simulink model "Test_OmniTorque_Lib"  (Simulink 7.6)
settings: Solver=ode3  StartTime=0.0  StopTime=inf  RelTol=1e-3
libraries: PhanTorque_3Dof_Library_32Bits x6
settings Model: Creator=carlos.aldana  LastModifiedBy=carlos.aldana
settings DebuggingCC: CheckSSInitialOutputMsg=off

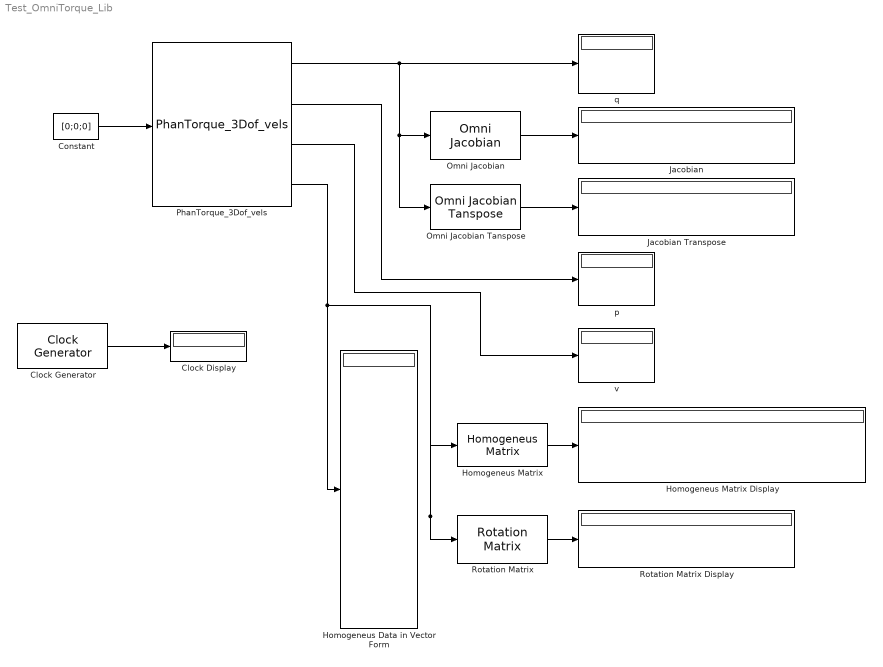
== system Test_OmniTorque_Lib ==
  Clock Display : Display
  Clock Generator : PhanTorque_3Dof_Library_32Bits/Clock Generator
  Constant : Constant  Value=[0;0;0]
  Homogeneus Data in Vector Form : Display
  Homogeneus Matrix : PhanTorque_3Dof_Library_32Bits/Homogeneus Matrix  SystemSampleTime=-1
  Homogeneus Matrix Display : Display
  Jacobian : Display
  Jacobian Transpose : Display
  Omni Jacobian : PhanTorque_3Dof_Library_32Bits/Omni Jacobian  SystemSampleTime=-1
  Omni Jacobian Tanspose : PhanTorque_3Dof_Library_32Bits/Omni Jacobian Tanspose  SystemSampleTime=-1
  PhanTorque_3Dof_vels : PhanTorque_3Dof_Library_32Bits/PhanTorque_3Dof_vels  Haptic_Name='Default PHANToM'
  Rotation Matrix : PhanTorque_3Dof_Library_32Bits/Rotation Matrix  SystemSampleTime=-1
  Rotation Matrix Display : Display
  p : Display
  q : Display
  v : Display
  wires:
  PhanTorque_3Dof_vels/4 -> Homogeneus Data in Vector Form/1, Homogeneus Matrix/1, Rotation Matrix/1
  PhanTorque_3Dof_vels/2 -> p/1
  PhanTorque_3Dof_vels/1 -> q/1, Omni Jacobian/1, Omni Jacobian Tanspose/1
  Omni Jacobian/1 -> Jacobian/1
  Rotation Matrix/1 -> Rotation Matrix Display/1
  Homogeneus Matrix/1 -> Homogeneus Matrix Display/1
  Clock Generator/1 -> Clock Display/1
  Omni Jacobian Tanspose/1 -> Jacobian Transpose/1
  PhanTorque_3Dof_vels/3 -> v/1
  Constant/1 -> PhanTorque_3Dof_vels/1
